simulink model "pendule_inv_capteur_etu"  (R2019a)
settings: Solver=ode45  StartTime=0.0  StopTime=tf  FixedStep=5  RelTol=1e-3
undefined symbols (not defined in the file): g, K, l, ue, xe
settings Model: Creator=nfoin  LastModifiedBy=nfoin

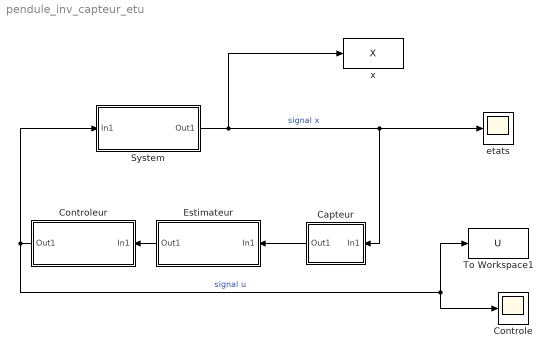
== system pendule_inv_capteur_etu ==
  Capteur : Subsystem
  Controle : Scope
  Controleur : Subsystem
  Estimateur : Subsystem
  System : Subsystem
  To Workspace1 : ToWorkspace  VariableName=U  SaveFormat=Timeseries  SampleTime=-1
  etats : Scope
  x : ToWorkspace  VariableName=X  SaveFormat=Timeseries  SampleTime=-1
  wires:
  System/1(Out1) -> x/1, etats/1, Capteur/1(In1)  "signal x"
  Controleur/1(Out1) -> System/1(In1), To Workspace1/1, Controle/1  "signal u"
  Capteur/1(Out1) -> Estimateur/1(In1)
  Estimateur/1(Out1) -> Controleur/1(In1)

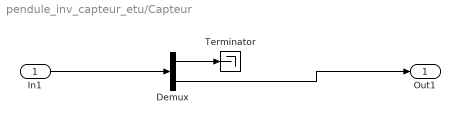
== system pendule_inv_capteur_etu/Capteur ==
  In1 : Inport
  Demux : Demux  Outputs=2
  Terminator : Terminator
  Out1 : Outport
  wires:
  In1/1 -> Demux/1
  Demux/1 -> Terminator/1
  Demux/2 -> Out1/1

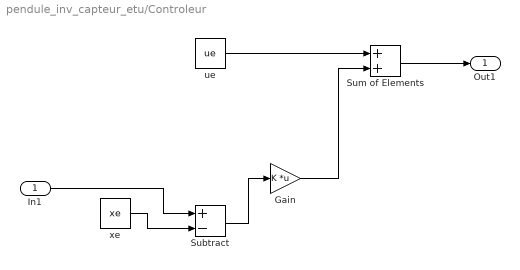
== system pendule_inv_capteur_etu/Controleur ==
  In1 : Inport
  Gain : Gain  Gain=K  Multiplication=Matrix(K*u)
  Subtract : Sum  Inputs=+-
  Sum of Elements : Sum
  ue : Constant  Value=ue
  xe : Constant  Value=xe
  Out1 : Outport
  wires:
  ue/1 -> Sum of Elements/1
  In1/1 -> Subtract/1
  xe/1 -> Subtract/2
  Subtract/1 -> Gain/1
  Gain/1 -> Sum of Elements/2
  Sum of Elements/1 -> Out1/1

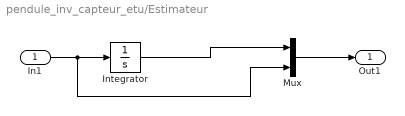
== system pendule_inv_capteur_etu/Estimateur ==
  In1 : Inport
  Integrator : Integrator  InitialCondition=-1
  Mux : Mux  Inputs=2
  Out1 : Outport
  wires:
  In1/1 -> Mux/2, Integrator/1
  Integrator/1 -> Mux/1
  Mux/1 -> Out1/1

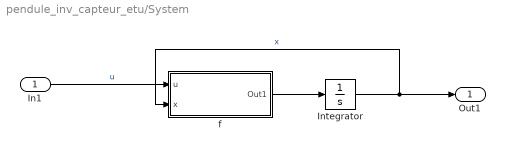
== system pendule_inv_capteur_etu/System ==
  In1 : Inport
  Integrator : Integrator
  f : Subsystem
  Out1 : Outport
  wires:
  In1/1 -> f/1(u)  "u"
  f/1(Out1) -> Integrator/1
  Integrator/1 -> f/2(x), Out1/1  "x"

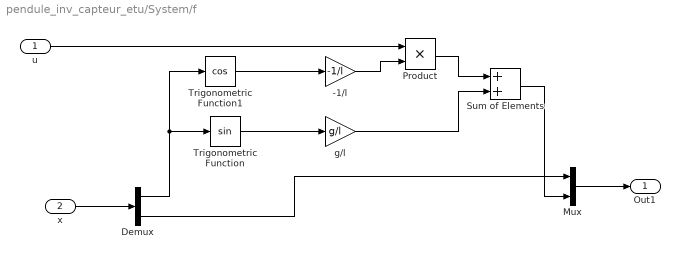
== system pendule_inv_capteur_etu/System/f ==
  u : Inport
  x : Inport  Port=2
  -1/l : Gain  Gain=-1/l
  Demux : Demux  Outputs=2
  Mux : Mux  Inputs=2
  Product : Product
  Sum of Elements : Sum
  Trigonometric Function : Trigonometry
  Trigonometric Function1 : Trigonometry  Operator=cos
  g/l : Gain  Gain=g/l
  Out1 : Outport
  wires:
  x/1 -> Demux/1
  Demux/1 -> Trigonometric Function1/1, Trigonometric Function/1
  Mux/1 -> Out1/1
  Trigonometric Function/1 -> g/l/1
  Demux/2 -> Mux/1
  Trigonometric Function1/1 -> -1/l/1
  -1/l/1 -> Product/2
  Product/1 -> Sum of Elements/1
  g/l/1 -> Sum of Elements/2
  u/1 -> Product/1
  Sum of Elements/1 -> Mux/2
